simulink model "dynctrl"  (R2020b)
settings: Solver=VariableStepAuto  StartTime=0.0  StopTime=20  RelTol=1e-3
values from neighbouring files (symbols this model uses):
  d = [b1 r2]    [dynamic_script.m]
  eta = 70    [dynamic_script.m]
  g = 9.81    [dynamic_script.m]
  J = [Je Ja]    [dynamic_script.m]
  Ke = 0.00767    [dynamic_script.m]
  Kt = 0.00767    [dynamic_script.m]
  l = [l1 l2]    [dynamic_script.m]
  La = 0.18    [dynamic_script.m]
  m = [m1 m2]    [dynamic_script.m]
  motor_switch = 1    [dynamic_script.m]
  qdot0 = [0;0]    [dynamic_script.m]
  Ra = 2.6    [dynamic_script.m]
  Vin = 0    [dynamic_script.m]
settings Model: Creator=lucas  LastModifiedBy=lucas

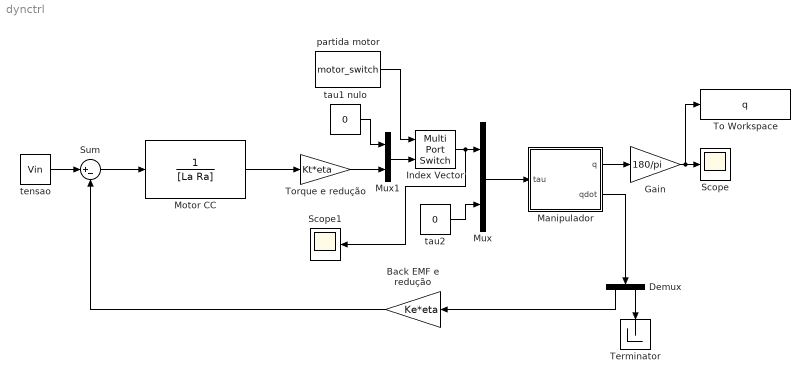
== system dynctrl ==
  Back EMF e redução : Gain  Gain=Ke*eta
  Demux : Demux  Outputs=2
  Gain : Gain  Gain=180/pi
  Index Vector : MultiPortSwitch  DataPortOrder=Zero-based contiguous  Inputs=1  zeroidx=on
  Manipulador : Subsystem
  Motor CC : TransferFcn  Denominator=[La Ra]
  Mux : Mux  Inputs=2
  Mux1 : Mux  Inputs=2
  Scope : Scope
  Scope1 : Scope
  Sum : Sum  Inputs=|+-
  Terminator : Terminator
  To Workspace : ToWorkspace  VariableName=q  SaveFormat=Timeseries  SampleTime=-1
  Torque e redução : Gain  Gain=Kt*eta
  partida motor : Constant  Value=motor_switch
  tau1 nulo : Constant  Value=0
  tau2 : Constant  Value=0
  tensao : Constant  Value=Vin
  wires:
  Manipulador/1(q) -> Gain/1
  tau2/1 -> Mux/2
  Mux/1 -> Manipulador/1(tau)
  Motor CC/1 -> Torque e redução/1
  Index Vector/1 -> Scope1/1, Mux/1
  Mux1/1 -> Index Vector/2
  tau1 nulo/1 -> Mux1/1
  Torque e redução/1 -> Mux1/2
  tensao/1 -> Sum/1
  Sum/1 -> Motor CC/1
  Manipulador/2(qdot) -> Demux/1
  Back EMF e redução/1 -> Sum/2
  partida motor/1 -> Index Vector/1
  Demux/1 -> Back EMF e redução/1
  Demux/2 -> Terminator/1
  Gain/1 -> To Workspace/1, Scope/1

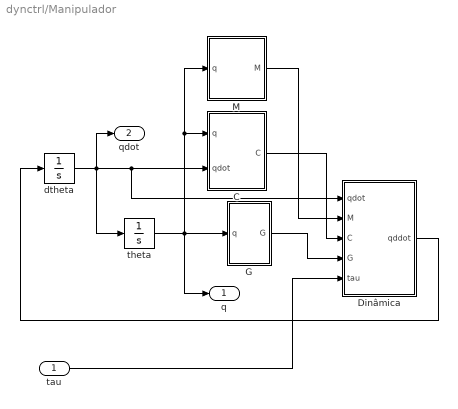
== system dynctrl/Manipulador ==
  tau : Inport
  C : Subsystem
  Dinâmica : MATLAB Function  TreatAsAtomicUnit=on
  G : Subsystem
  M : Subsystem
  dtheta : Integrator  InitialCondition=qdot0
  theta : Integrator  InitialCondition=[0;pi/2-0.01]
  q : Outport
  qdot : Outport  Port=2
  wires:
  C/1(C) -> Dinâmica/3(C)
  dtheta/1 -> qdot/1, Dinâmica/1(qdot), C/2(qdot), theta/1
  theta/1 -> q/1, M/1(q), C/1(q), G/1(q)
  M/1(M) -> Dinâmica/2(M)
  tau/1 -> Dinâmica/5(tau)
  Dinâmica/1(qddot) -> dtheta/1
  G/1(G) -> Dinâmica/4(G)

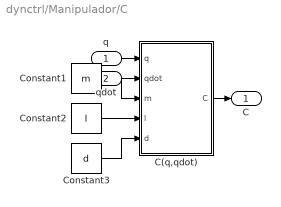
== system dynctrl/Manipulador/C ==
  q : Inport
  qdot : Inport  Port=2
  C(q,qdot) : MATLAB Function  TreatAsAtomicUnit=on
  Constant1 : Constant  Value=m
  Constant2 : Constant  Value=l
  Constant3 : Constant  Value=d
  C : Outport
  wires:
  C(q,qdot)/1(C) -> C/1
  Constant2/1 -> C(q,qdot)/4(l)
  qdot/1 -> C(q,qdot)/2(qdot)
  Constant3/1 -> C(q,qdot)/5(d)
  Constant1/1 -> C(q,qdot)/3(m)
  q/1 -> C(q,qdot)/1(q)

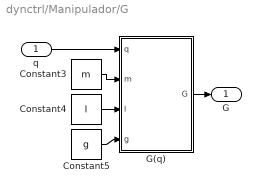
== system dynctrl/Manipulador/G ==
  q : Inport
  Constant3 : Constant  Value=m
  Constant4 : Constant  Value=l
  Constant5 : Constant  Value=g
  G(q) : MATLAB Function  TreatAsAtomicUnit=on
  G : Outport
  wires:
  Constant4/1 -> G(q)/3(l)
  G(q)/1(G) -> G/1
  Constant3/1 -> G(q)/2(m)
  Constant5/1 -> G(q)/4(g)
  q/1 -> G(q)/1(q)

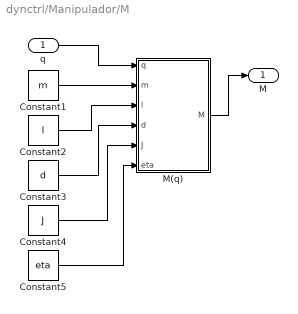
== system dynctrl/Manipulador/M ==
  q : Inport
  Constant1 : Constant  Value=m
  Constant2 : Constant  Value=l
  Constant3 : Constant  Value=d
  Constant4 : Constant  Value=J
  Constant5 : Constant  Value=eta
  M(q) : MATLAB Function  TreatAsAtomicUnit=on
  M : Outport
  wires:
  Constant3/1 -> M(q)/4(d)
  Constant2/1 -> M(q)/3(l)
  Constant1/1 -> M(q)/2(m)
  M(q)/1(M) -> M/1
  q/1 -> M(q)/1(q)
  Constant4/1 -> M(q)/5(J)
  Constant5/1 -> M(q)/6(eta)

== matlab function dynctrl/Manipulador/C/C(q,qdot) ==
  data: q input; qdot input; C output; m input; l input; d input
function C = fcn(q,qdot,m,l,d)
    q1 = q(1);
    q2 = q(2);
    
    q1dot = qdot(1);
    q2dot = qdot(2);
    
    m1 = m(1);
    m2 = m(2);
    
    l1 = l(1);
    l2 = l(2);
    
    b1 = d(1);
    r2 = d(2);
    
    C11 = 0;
    C12 = (m2*sin(2*q2)*(4*l2^2 - 3*r2^2)*q1dot)/12 + 0.5*l1*l2*m2*sin(q2)*q2dot;
    C21 = -(m2*sin(2*q2)*(4*l2^2 - 3*r2^2)*q1dot)/24 - (l1*l2*m2*sin(q2)*q2dot)/4;
    C22 = (l1*l2*m2*sin(q2)*q1dot)/4;
    
    C = [C11 C12;
        C21 C22];
end

== matlab function dynctrl/Manipulador/M/M(q) ==
  data: q input; M output; m input; l input; d input; J input; eta input
function M = fcn(q,m,l,d, J, eta)
    q1 = q(1);
    q2 = q(2);
    
    m1 = m(1);
    m2 = m(2);
    
    l1 = l(1);
    l2 = l(2);
    
    b1 = d(1);
    r2 = d(2);
    
    Je = J(1);
    Ja = J(2);
    
    B11 = (m1*(l1^2 + b1^2))/12  +  m1*(l1/2)^2 + m2*l1^2 +(m2*l2^2*sin(q2)^2)/4 + (m2*3*r2^2 + l2^2*sin(q2)^2 + 3*r2^2*cos(q2)^2)/12;
    B11_motor = Je+(eta^2)*Ja;
    B12 = -((l1*l2*m2)*cos(q2))/2;
    B21 = B12;
    B22 = m2*(l2/2)^2 + (m2*(3*r2^2 + l2^2))/12;
    M = [B11+B11_motor B12;B21 B22];
end

== matlab function dynctrl/Manipulador/G/G(q) ==
  data: q input; G output; m input; l input; g input
function G = fcn(q,m,l,g)
    q1 = q(1);
    q2 = q(2);
    
    m1 = m(1);
    m2 = m(2);
    
    l1 = l(1);
    l2 = l(2);

    G1 = 0;
    G2 = -0.5*m2*g*l2*sin(q2);
    
    G = [G1;
        G2];
end

== matlab function dynctrl/Manipulador/Dinâmica ==
  data: qddot output; qdot input; M input; C input; G input; tau input
function qddot = fcn(qdot,M,C,G,tau)
    qddot = -inv(M)*(C*qdot+G-tau);
end
